simulink model "Par_model_sim_CHB9"  (R2023b)
settings: Solver=FixedStepAuto  StartTime=0.0  StopTime=5  FixedStep=1e-6  RelTol=1e-3
InitFcn:
  | sysinit
values from neighbouring files (symbols this model uses):
  C = 0.0234    [sysinit.m]
  f_out = frequency_out_start : frequency_out_interval : frequency_out_end    [simout_chb_par.m]    (also in simout_chbjt_par.m = frequency_modulate_start : frequency_modulate_interval : fre)
  f_switch = 250    [sysinit.m]
  fn = 50    [sysinit.m]
  L = 0.002    [sysinit.m]
  L_ori = 0.02    [sysinit.m]
  L_sec = 0.06    [sysinit.m]
  m_par = modulate_radio_start : modulate_radio_interval : modulate_radio_end    [simout_chb_par.m]
  P0 = 8e6    (= 8000000)    [sysinit.m]
  R = 1.5    [sysinit.m]
  Source_Amp = 10000    [sysinit.m]
  st = 1e-6    (= 1e-06)    [sysinit.m]
  Td = 15e-7    (= 1.5e-06)    [sysinit.m]
  Ul_in = 1900    [sysinit.m]
libraries: spsSeriesRLCBranchLib x123, spsDiodeLib x60, spsIGBTLib x48, spsCurrentMeasurementLib x16, spsThreePhaseVIMeasurementLib x13, spsOnDelayLib x12, spsUniversalBridgeLib x12, spsMultiWindingTransformerLib x9, simulink x3, spsVoltageMeasurementLib x3, spsRMSLib x2, spsThreePhaseProgrammableVoltageSourceLib x1
(part 3 of 3)

== system Par_model_sim_CHB9/Subsystem3 ==
  Multi-Winding Transformer10 : spsMultiWindingTransformerLib/Multi-Winding Transformer  LeftWindings=1  RightWindings=6  TappedWindings=no taps  NumberOfTaps=2  SetSaturation=off  Hysteresis=off  DataFile='hysteresis.mat'  Measurements=None  UNITS=pu  NominalPower=[P0 fn]  NominalVoltages="[ Source_Amp  Ul_in 0.366/3.721*Source_Amp*(1-0.366)/0.366 0.366/3.721*Source_Amp Ul_in*sqrt(3) 0.366/3.721*Source_Amp*(1-0.366)/0.366 0.366/3.721*Source_Amp]"  WindingResistances="[ 0.005   0.005 0.005 0.005  0.005  0.005  0.005]"  WindingInductances="[ L_ori*6  L_sec L_sec L_sec L_sec L_sec L_sec]"  Rm=50  Lm=50  Saturation=[ 0,0 ; 0.0024,1.2 ; 1.0,1.52 ]  SpecifyInitialFlux=off  InitialFlux=0  BreakLoop=off  DiscreteSolver=Trapezoidal iterative  DataType=off  TransfoNumber=1
      settings: LibrarySourceBlock=|
      | sps_lib/Power Grid Elements/Multi-Winding
      | Transformer
  Multi-Winding Transformer11 : spsMultiWindingTransformerLib/Multi-Winding Transformer  LeftWindings=1  RightWindings=6  TappedWindings=no taps  NumberOfTaps=2  SetSaturation=off  Hysteresis=off  DataFile='hysteresis.mat'  Measurements=None  UNITS=pu  NominalPower=[P0 fn]  NominalVoltages="[ Source_Amp  Ul_in 0.366/3.721*Source_Amp*(1-0.366)/0.366 0.366/3.721*Source_Amp Ul_in*sqrt(3) 0.366/3.721*Source_Amp*(1-0.366)/0.366 0.366/3.721*Source_Amp]"  WindingResistances="[ 0.005   0.005 0.005 0.005  0.005  0.005  0.005]"  WindingInductances="[ L_ori*6  L_sec L_sec L_sec L_sec L_sec L_sec]"  Rm=50  Lm=50  Saturation=[ 0,0 ; 0.0024,1.2 ; 1.0,1.52 ]  SpecifyInitialFlux=off  InitialFlux=0  BreakLoop=off  DiscreteSolver=Trapezoidal iterative  DataType=off  TransfoNumber=1
      settings: LibrarySourceBlock=|
      | sps_lib/Power Grid Elements/Multi-Winding
      | Transformer
  Multi-Winding Transformer9 : spsMultiWindingTransformerLib/Multi-Winding Transformer  LeftWindings=1  RightWindings=6  TappedWindings=no taps  NumberOfTaps=2  SetSaturation=off  Hysteresis=off  DataFile='hysteresis.mat'  Measurements=None  UNITS=pu  NominalPower=[P0 fn]  NominalVoltages="[ Source_Amp  Ul_in 0.366/3.721*Source_Amp*(1-0.366)/0.366 0.366/3.721*Source_Amp Ul_in*sqrt(3) 0.366/3.721*Source_Amp*(1-0.366)/0.366 0.366/3.721*Source_Amp]"  WindingResistances="[ 0.005   0.005 0.005 0.005  0.005  0.005  0.005]"  WindingInductances=[ L_ori*6 L_sec L_sec L_sec L_sec L_sec L_sec ]/6  Rm=50  Lm=50  Saturation=[ 0,0 ; 0.0024,1.2 ; 1.0,1.52 ]  SpecifyInitialFlux=off  InitialFlux=0  BreakLoop=off  DiscreteSolver=Trapezoidal iterative  DataType=off  TransfoNumber=1
      settings: LibrarySourceBlock=|
      | sps_lib/Power Grid Elements/Multi-Winding
      | Transformer
  1+ : PMIOPort  Side=Left
  1+1 : PMIOPort  Port=2  Side=Left
  1+2 : PMIOPort  Port=3  Side=Left
  p-15a : PMIOPort  Port=4  Side=Right
  p-15b : PMIOPort  Port=5  Side=Right
  p-15c : PMIOPort  Port=6  Side=Right
  p0a : PMIOPort  Port=7  Side=Right
  p0b : PMIOPort  Port=8  Side=Right
  p0c : PMIOPort  Port=9  Side=Right
  p15a : PMIOPort  Port=10  Side=Right
  p15b : PMIOPort  Port=11  Side=Right
  p15c : PMIOPort  Port=12  Side=Right
  p30a : PMIOPort  Port=13  Side=Right
  p30b : PMIOPort  Port=14  Side=Right
  p30c : PMIOPort  Port=15  Side=Right
  connections:
  Multi-Winding Transformer11/LConn1 -- 1+2/RConn1
  p15c/RConn1 -- Multi-Winding Transformer11/RConn11
  p15a/RConn1 -- Multi-Winding Transformer9/RConn11
  p0c/RConn1 -- Multi-Winding Transformer11/RConn1
  Multi-Winding Transformer10/LConn1 -- 1+1/RConn1
  p15b/RConn1 -- Multi-Winding Transformer10/RConn11
  p30b/RConn1 -- Multi-Winding Transformer10/RConn7 -- Multi-Winding Transformer11/RConn8
  p0a/RConn1 -- Multi-Winding Transformer9/RConn1
  Multi-Winding Transformer9/LConn1 -- 1+/RConn1
  Multi-Winding Transformer11/RConn10 -- Multi-Winding Transformer10/RConn12 -- Multi-Winding Transformer10/RConn9
  p30c/RConn1 -- Multi-Winding Transformer11/RConn7 -- Multi-Winding Transformer9/RConn8
  Multi-Winding Transformer9/RConn6 -- Multi-Winding Transformer9/RConn3 -- Multi-Winding Transformer11/RConn4
  p30a/RConn1 -- Multi-Winding Transformer9/RConn7 -- Multi-Winding Transformer10/RConn8
  Multi-Winding Transformer11/RConn6 -- Multi-Winding Transformer10/RConn4 -- Multi-Winding Transformer11/RConn3
  Multi-Winding Transformer10/RConn3 -- Multi-Winding Transformer9/RConn4 -- Multi-Winding Transformer10/RConn6
  Multi-Winding Transformer10/RConn1 -- p0b/RConn1
  Multi-Winding Transformer10/RConn10 -- Multi-Winding Transformer9/RConn9 -- Multi-Winding Transformer9/RConn12
  p-15b/RConn1 -- Multi-Winding Transformer10/RConn5
  p-15c/RConn1 -- Multi-Winding Transformer11/RConn5
  Multi-Winding Transformer9/RConn10 -- Multi-Winding Transformer11/RConn9 -- Multi-Winding Transformer11/RConn12
  p-15a/RConn1 -- Multi-Winding Transformer9/RConn5
  Multi-Winding Transformer9/LConn2 -- Multi-Winding Transformer10/LConn2 -- Multi-Winding Transformer11/LConn2
  Multi-Winding Transformer10/RConn2 -- Multi-Winding Transformer9/RConn2 -- Multi-Winding Transformer11/RConn2

== system Par_model_sim_CHB9/Subsystem4 ==
  Current Measurement : spsCurrentMeasurementLib/Current Measurement  PhasorSimulation=off  OutputType=Complex  PSBequivalent=0
  Voltage Measurement : spsVoltageMeasurementLib/Voltage Measurement  PhasorSimulation=off  OutputType=Complex  PSBequivalent=0
  + : PMIOPort  Side=Left
  - : PMIOPort  Port=2  Side=Left
  +OUT : PMIOPort  Port=3  Side=Right
  -OUT : PMIOPort  Port=4  Side=Right
  tag scope: Idc=global, Udc=global
  wires:
  Current Measurement/1 -> [Idc]
  Voltage Measurement/1 -> [Udc]
  connections:
  Current Measurement/RConn1 -- +OUT/RConn1
  -/RConn1 -- -OUT/RConn1 -- Voltage Measurement/LConn2
  +/RConn1 -- Current Measurement/LConn1 -- Voltage Measurement/LConn1

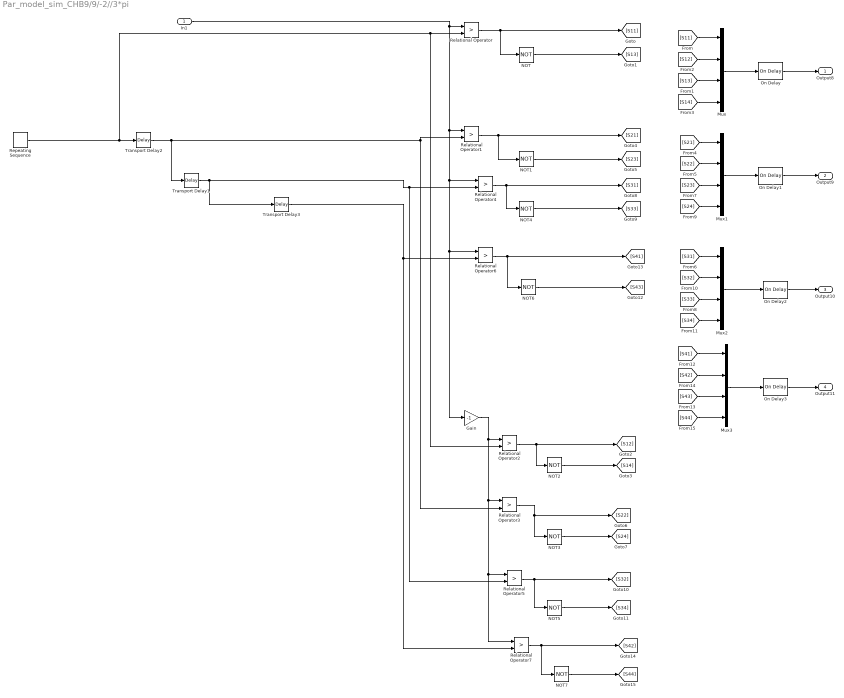
== system Par_model_sim_CHB9/9/-2//3*pi ==
  In1 : Inport
  Gain : Gain  Gain=-1
  Mux{,1..3} (4 alike) : Mux
  NOT{,1..7} (8 alike) : Logic  Operator=NOT  AllPortsSameDT=off  OutDataTypeStr=boolean
  On Delay{,1..3} (4 alike) : spsOnDelayLib/On Delay  DelayType=On delay  delay=ttd  ic=0  Ts=0
  Relational Operator{,1..7} (8 alike) : RelationalOperator  Operator=>  OutDataTypeStr=boolean  RndMeth=Simplest  InputSameDT=off
  Repeating Sequence : simulink/Sources/Repeating Sequence  rep_seq_t=[0 0.5 1]/f_car  rep_seq_y=[-1 1 -1]*1000
  Transport Delay1 : TransportDelay  DelayTime=tt/f_car  BufferSize=3072
  Transport Delay2 : TransportDelay  DelayTime=tt/f_car  BufferSize=3072
  Transport Delay3 : TransportDelay  DelayTime=tt/f_car  BufferSize=3072
  Output8 : Outport
  Output9 : Outport  Port=2
  Output10 : Outport  Port=3
  Output11 : Outport  Port=4
  wires:
  On Delay2/1 -> Output10/1
  On Delay1/1 -> Output9/1
  On Delay/1 -> Output8/1
  NOT/1 -> [S13]
  Transport Delay1/1 -> Relational Operator5/2, Relational Operator4/2, Transport Delay3/1
  Transport Delay2/1 -> Transport Delay1/1, Relational Operator3/2, Relational Operator1/2
  [S14] -> Mux/4
  [S23] -> Mux1/3
  [S12] -> Mux/2
  In1/1 -> Relational Operator4/1, Relational Operator6/1, Gain/1, Relational Operator1/1, Relational Operator/1
  [S34] -> Mux2/4
  [S32] -> Mux2/2
  Mux2/1 -> On Delay2/1
  Relational Operator5/1 -> [S32], NOT5/1
  NOT2/1 -> [S14]
  [S21] -> Mux1/1
  NOT4/1 -> [S33]
  Relational Operator1/1 -> NOT1/1, [S21]
  [S22] -> Mux1/2
  [S33] -> Mux2/3
  NOT3/1 -> [S24]
  Mux/1 -> On Delay/1
  Repeating Sequence/1 -> Relational Operator2/2, Relational Operator/2, Transport Delay2/1
  [S24] -> Mux1/4
  Relational Operator4/1 -> [S31], NOT4/1
  Gain/1 -> Relational Operator7/1, Relational Operator5/1, Relational Operator3/1, Relational Operator2/1
  [S13] -> Mux/3
  Relational Operator2/1 -> NOT2/1, [S12]
  [S31] -> Mux2/1
  [S11] -> Mux/1
  NOT5/1 -> [S34]
  Relational Operator/1 -> NOT/1, [S11]
  NOT1/1 -> [S23]
  Mux1/1 -> On Delay1/1
  Relational Operator3/1 -> [S22], NOT3/1
  Relational Operator6/1 -> [S41], NOT6/1
  NOT6/1 -> [S43]
  [S41] -> Mux3/1
  [S43] -> Mux3/3
  Mux3/1 -> On Delay3/1
  On Delay3/1 -> Output11/1
  NOT7/1 -> [S44]
  Relational Operator7/1 -> NOT7/1, [S42]
  Transport Delay3/1 -> Relational Operator7/2, Relational Operator6/2
  [S42] -> Mux3/2
  [S44] -> Mux3/4

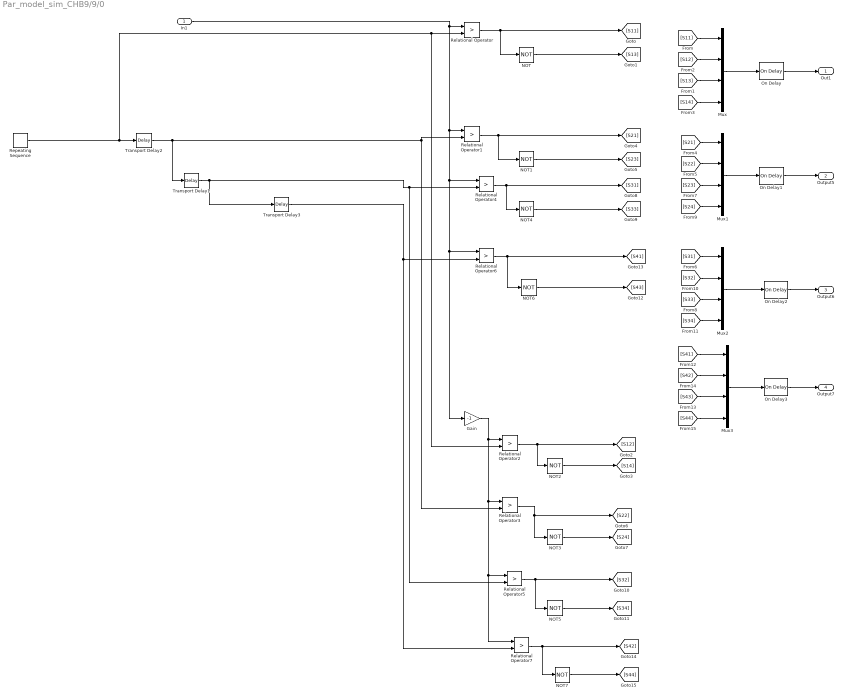
== system Par_model_sim_CHB9/9/0 ==
  In1 : Inport
  Gain : Gain  Gain=-1
  Mux{,1..3} (4 alike) : Mux
  NOT{,1..7} (8 alike) : Logic  Operator=NOT  AllPortsSameDT=off  OutDataTypeStr=boolean
  On Delay{,1..3} (4 alike) : spsOnDelayLib/On Delay  DelayType=On delay  delay=ttd  ic=0  Ts=0
  Relational Operator{,1..7} (8 alike) : RelationalOperator  Operator=>  OutDataTypeStr=boolean  RndMeth=Simplest  InputSameDT=off
  Repeating Sequence : simulink/Sources/Repeating Sequence  rep_seq_t=[0 0.5 1]/f_car  rep_seq_y=[-1 1 -1]*1000
  Transport Delay1 : TransportDelay  DelayTime=tt/f_car  BufferSize=3072
  Transport Delay2 : TransportDelay  DelayTime=tt/f_car  BufferSize=3072
  Transport Delay3 : TransportDelay  DelayTime=tt/f_car  BufferSize=3072
  Out1 : Outport
  Output5 : Outport  Port=2
  Output6 : Outport  Port=3
  Output7 : Outport  Port=4
  wires:
  On Delay2/1 -> Output6/1
  On Delay1/1 -> Output5/1
  On Delay/1 -> Out1/1
  NOT/1 -> [S13]
  Transport Delay1/1 -> Relational Operator5/2, Relational Operator4/2, Transport Delay3/1
  Transport Delay2/1 -> Transport Delay1/1, Relational Operator3/2, Relational Operator1/2
  [S14] -> Mux/4
  [S23] -> Mux1/3
  [S12] -> Mux/2
  In1/1 -> Relational Operator4/1, Relational Operator6/1, Gain/1, Relational Operator1/1, Relational Operator/1
  [S34] -> Mux2/4
  [S32] -> Mux2/2
  Mux2/1 -> On Delay2/1
  Relational Operator5/1 -> [S32], NOT5/1
  NOT2/1 -> [S14]
  [S21] -> Mux1/1
  NOT4/1 -> [S33]
  Relational Operator1/1 -> NOT1/1, [S21]
  [S22] -> Mux1/2
  [S33] -> Mux2/3
  NOT3/1 -> [S24]
  Mux/1 -> On Delay/1
  Repeating Sequence/1 -> Relational Operator2/2, Relational Operator/2, Transport Delay2/1
  [S24] -> Mux1/4
  Relational Operator4/1 -> [S31], NOT4/1
  Gain/1 -> Relational Operator7/1, Relational Operator5/1, Relational Operator3/1, Relational Operator2/1
  [S13] -> Mux/3
  Relational Operator2/1 -> NOT2/1, [S12]
  [S31] -> Mux2/1
  [S11] -> Mux/1
  NOT5/1 -> [S34]
  Relational Operator/1 -> NOT/1, [S11]
  NOT1/1 -> [S23]
  Mux1/1 -> On Delay1/1
  Relational Operator3/1 -> [S22], NOT3/1
  Relational Operator6/1 -> [S41], NOT6/1
  NOT6/1 -> [S43]
  [S41] -> Mux3/1
  [S43] -> Mux3/3
  Mux3/1 -> On Delay3/1
  On Delay3/1 -> Output7/1
  NOT7/1 -> [S44]
  Relational Operator7/1 -> NOT7/1, [S42]
  Transport Delay3/1 -> Relational Operator7/2, Relational Operator6/2
  [S42] -> Mux3/2
  [S44] -> Mux3/4

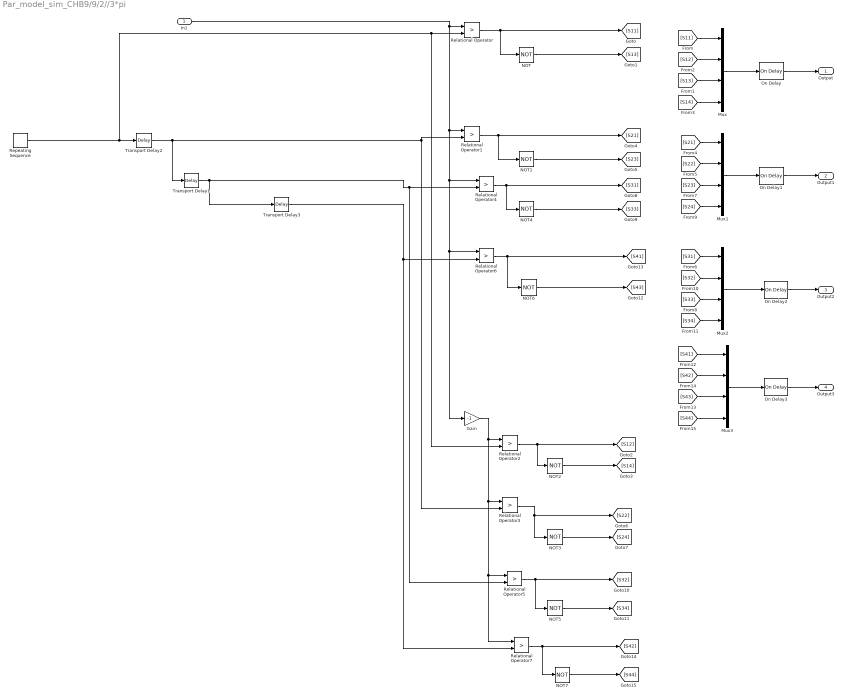
== system Par_model_sim_CHB9/9/2//3*pi ==
  In1 : Inport
  Gain : Gain  Gain=-1
  Mux{,1..3} (4 alike) : Mux
  NOT{,1..7} (8 alike) : Logic  Operator=NOT  AllPortsSameDT=off  OutDataTypeStr=boolean
  On Delay{,1..3} (4 alike) : spsOnDelayLib/On Delay  DelayType=On delay  delay=ttd  ic=0  Ts=0
  Relational Operator{,1..7} (8 alike) : RelationalOperator  Operator=>  OutDataTypeStr=boolean  RndMeth=Simplest  InputSameDT=off
  Repeating Sequence : simulink/Sources/Repeating Sequence  rep_seq_t=[0 0.5 1]/f_car  rep_seq_y=[-1 1 -1]*1000
  Transport Delay1 : TransportDelay  DelayTime=tt/f_car  BufferSize=3072
  Transport Delay2 : TransportDelay  DelayTime=tt/f_car  BufferSize=3072
  Transport Delay3 : TransportDelay  DelayTime=tt/f_car  BufferSize=3072
  Output : Outport
  Output1 : Outport  Port=2
  Output2 : Outport  Port=3
  Output3 : Outport  Port=4
  wires:
  On Delay2/1 -> Output2/1
  On Delay1/1 -> Output1/1
  On Delay/1 -> Output/1
  NOT/1 -> [S13]
  Transport Delay1/1 -> Relational Operator5/2, Relational Operator4/2, Transport Delay3/1
  Transport Delay2/1 -> Transport Delay1/1, Relational Operator3/2, Relational Operator1/2
  [S14] -> Mux/4
  [S23] -> Mux1/3
  [S12] -> Mux/2
  In1/1 -> Relational Operator4/1, Relational Operator6/1, Gain/1, Relational Operator1/1, Relational Operator/1
  [S34] -> Mux2/4
  [S32] -> Mux2/2
  Mux2/1 -> On Delay2/1
  Relational Operator5/1 -> [S32], NOT5/1
  NOT2/1 -> [S14]
  [S21] -> Mux1/1
  NOT4/1 -> [S33]
  Relational Operator1/1 -> NOT1/1, [S21]
  [S22] -> Mux1/2
  [S33] -> Mux2/3
  NOT3/1 -> [S24]
  Mux/1 -> On Delay/1
  Repeating Sequence/1 -> Relational Operator2/2, Relational Operator/2, Transport Delay2/1
  [S24] -> Mux1/4
  Relational Operator4/1 -> [S31], NOT4/1
  Gain/1 -> Relational Operator7/1, Relational Operator5/1, Relational Operator3/1, Relational Operator2/1
  [S13] -> Mux/3
  Relational Operator2/1 -> NOT2/1, [S12]
  [S31] -> Mux2/1
  [S11] -> Mux/1
  NOT5/1 -> [S34]
  Relational Operator/1 -> NOT/1, [S11]
  NOT1/1 -> [S23]
  Mux1/1 -> On Delay1/1
  Relational Operator3/1 -> [S22], NOT3/1
  Relational Operator6/1 -> [S41], NOT6/1
  NOT6/1 -> [S43]
  [S41] -> Mux3/1
  [S43] -> Mux3/3
  Mux3/1 -> On Delay3/1
  On Delay3/1 -> Output3/1
  NOT7/1 -> [S44]
  Relational Operator7/1 -> NOT7/1, [S42]
  Transport Delay3/1 -> Relational Operator7/2, Relational Operator6/2
  [S42] -> Mux3/2
  [S44] -> Mux3/4

== system Par_model_sim_CHB9/9/Subsystem ==
  In1 : Inport
  In2 : Inport  Port=2
  In3 : Inport  Port=3
  Add{1..3,9} (4 alike) : Sum
  Gain : Gain  Gain=-0.5
  Max : MinMax  Function=max  Inputs=3
  Max1 : MinMax  Inputs=3
  Out1 : Outport
  Out2 : Outport  Port=2
  Out3 : Outport  Port=3
  wires:
  Add3/1 -> Out2/1
  Add2/1 -> Out1/1
  Add9/1 -> Out3/1
  Add1/1 -> Gain/1
  Max1/1 -> Add1/2
  Max/1 -> Add1/1
  Gain/1 -> Add2/1, Add3/1, Add9/1
  In1/1 -> Max/1, Add2/2, Max1/1
  In3/1 -> Max/3, Max1/3, Add9/2
  In2/1 -> Max/2, Max1/2, Add3/2
